simulink model "P6_simulink"  (R2023a)
settings: Solver=ode23t  StartTime=0.0  StopTime=0.01  MaxStep=0.000001  RelTol=1e-3
values from neighbouring files (symbols this model uses):
  C = 0.1e-6    (= 1e-07)    [DobleP6.m]
  L = 4e-3    (= 0.004)    [DobleP6.m]
  R = 100    [DobleP6.m]
settings Model: Creator=mluser  LastModifiedBy=mluser
settings OptimizationCC: ReuseModelBlockBuffer=off

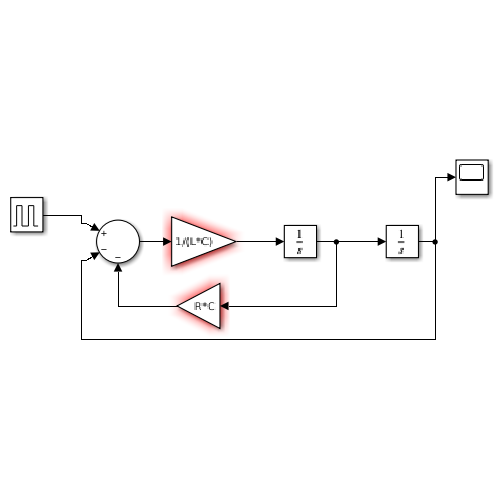
[thumbnail: Simulink's stored preview of the top-level diagram]
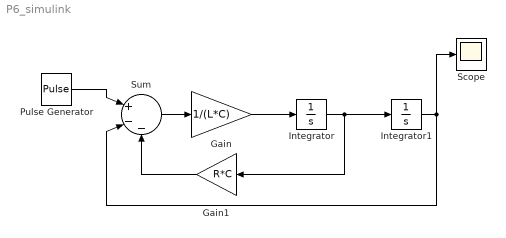
== system P6_simulink ==
  Gain : Gain  Gain=1/(L*C)
  Gain1 : Gain  Gain=R*C
  Integrator : Integrator
  Integrator1 : Integrator
  Pulse Generator : DiscretePulseGenerator  PulseType=Time based  Amplitude=5  Period=0.002  PulseWidth=50
  Scope : Scope
  Sum : Sum  Inputs=|+--
  wires:
  Gain1/1 -> Sum/3
  Integrator/1 -> Gain1/1, Integrator1/1
  Sum/1 -> Gain/1
  Gain/1 -> Integrator/1
  Integrator1/1 -> Scope/1, Sum/2
  Pulse Generator/1 -> Sum/1
